simulink model "BEML_EMU"  (R2019b)
settings: configuration reference "ConfigSet_SimIntegration" (kept outside this file)
model workspace (MAT data in the model file):
  BrakesSampleTime = 0.01
  ConfigSampleTime = 0.05
  CouplingSampleTime = 0.05
  DoorsSampleTime = 0.05
  DynamicsSampleTime = 0.001
  ElectricalSampleTime = 0.05
  PRM_SimIntegration = Simulink.Parameter
  PRM_SimIntegration.Value.Dynamics.SnapToZeroVelocity = 1e-05
  PRM_SimIntegration.Value.Brakes.Equipment.AxleBrakeConfig = [1; 1; 2; 2; 0; 0]
  PRM_SimIntegration.Value.Brakes.Equipment.AxleParkBrakeConfig = [1; 2; 3; 4; 0; 0]
  PRM_SimIntegration.Value.Brakes.Equipment.NumberOfBrakeCylindersPerAxle = 2
  PRM_SimIntegration.Value.Brakes.Equipment.BrakeShoeType : enumeration (value not decoded)
  PRM_SimIntegration.Value.Brakes.BrakeCylinder.BrakeCylinderPreload = 5000
  PRM_SimIntegration.Value.Brakes.BrakeCylinder.BrakeCylinderArea = 0.024
  PRM_SimIntegration.Value.Brakes.BrakeCylinder.BrakeBeamFactor = 4.35
  PRM_SimIntegration.Value.Brakes.BrakeCylinder.BrakeEfficiency = 95
  PRM_SimIntegration.Value.Brakes.BrakeDisc.DiscBrakeRatio = 0
  PRM_SimIntegration.Value.Brakes.BrakeDisc.DiscBrakeFrictionCoef = 0
  PRM_SimIntegration.Value.Brakes.BrakeFade.BrakeTemperatures = [273; 323; 373; 423; 473; 523; 573; 623; 673; 723]
  PRM_SimIntegration.Value.Brakes.BrakeFade.BrakeEfficiencies = [1; 1; 1; 1; 1; 1; 1; 1; 1; 1]
  PRM_SimIntegration.Value.Brakes.ThermalModel.BrakeInitialTemperature = 298
  PRM_SimIntegration.Value.Brakes.ThermalModel.BrakeSpecificHeat = 500
  PRM_SimIntegration.Value.Brakes.ThermalModel.BrakeEmissivity = 0.3
  PRM_SimIntegration.Value.Brakes.ThermalModel.BrakeThermalMass = 300
  PRM_SimIntegration.Value.Brakes.ParkBrakes.ParkBrakePressures = [380000 480000]
  PRM_SimIntegration.Value.Brakes.ParkBrakes.AxleParkBrakePistonForces = [31500 0]
  PRM_SimIntegration.Value.Pneumatics.BrakeControl.LoadCompensationGains = [0.66 1]
  PRM_SimIntegration.Value.Pneumatics.BrakeControl.MaxPressure = 443000
  PRM_SimIntegration.Value.Pneumatics.MainReservoir.ResetPressure = 1000000
  PRM_SimIntegration.Value.Pneumatics.MainReservoir.MaxPressure = 1200000
  PRM_SimIntegration.Value.Pneumatics.MainReservoir.Volume = 0.2
  PRM_SimIntegration.Value.Pneumatics.MainReservoir.SwitchONPressure = 1000000
  PRM_SimIntegration.Value.Pneumatics.MainReservoir.SwitchOFFPressure = 750000
  PRM_SimIntegration.Value.Pneumatics.MainReservoir.CompressorMassFlowRate = 0.022
  PRM_SimIntegration.Value.Pneumatics.MainReservoir.BlowOffONPressure = 1050000
  PRM_SimIntegration.Value.Pneumatics.MainReservoir.BlowOffOFFPressure = 1000000
  PRM_SimIntegration.Value.Pneumatics.MainReservoirPipe.ResetPressure = 1000000
  PRM_SimIntegration.Value.Pneumatics.MainReservoirPipe.SwitchONPressure = 1000000
  PRM_SimIntegration.Value.Pneumatics.MainReservoirPipe.SwitchOFFPressure = 750000
  PRM_SimIntegration.Value.Pneumatics.Sanding.SwitchONPressure = 380000
  PRM_SimIntegration.Value.Pneumatics.Sanding.SwitchOFFPressure = 360000
  PRM_SimIntegration.Value.Pneumatics.AirSuspension.LoadCompensationMasses = [21000 33350]
  PRM_SimIntegration.Value.Pneumatics.AirSuspension.LoadCompensationPressures = [165000 440000]
  PRM_SimIntegration.Value.Pneumatics.AirSuspension.MaxPressure = 510000
  PRM_SimIntegration.Value.Pneumatics.AirSuspension.Volume = 0.07
  PRM_SimIntegration.Value.Pneumatics.AirSuspension.SwitchONPressure = 220000
  PRM_SimIntegration.Value.Pneumatics.AirSuspension.SwitchOFFPressure = 180000
  PRM_SimIntegration.Value.Pneumatics.Horn.SwitchONPressure = 140000
  PRM_SimIntegration.Value.Pneumatics.AuxiliaryReservoir.ResetPressure = 1000000
  PRM_SimIntegration.Value.Pneumatics.AuxiliaryReservoir.MaxPressure = 1000000
  PRM_SimIntegration.Value.Pneumatics.AuxiliaryReservoir.Volume = 0.025
  PRM_SimIntegration.Value.Pneumatics.AuxiliaryReservoir.SwitchONPressure = 700000
  PRM_SimIntegration.Value.Pneumatics.AuxiliaryReservoir.SwitchOFFPressure = 600000
  PRM_SimIntegration.Value.Pneumatics.AuxiliaryReservoir.CompressorMassFlowRate = 0.0014
  PRM_SimIntegration.Value.Pneumatics.AuxiliaryReservoir.BlowOffONPressure = 1020000
  PRM_SimIntegration.Value.Pneumatics.AuxiliaryReservoir.BlowOffOFFPressure = 1000000
  PRM_SimIntegration.Value.Pneumatics.Pantograph.ResetPressure = 0
  PRM_SimIntegration.Value.Pneumatics.Pantograph.MaxPressure = 1000000
  PRM_SimIntegration.Value.Pneumatics.Pantograph.Volume = 0.003
  PRM_SimIntegration.Value.Pneumatics.Pantograph.SwitchONPressure = 380000
  PRM_SimIntegration.Value.Pneumatics.Pantograph.SwitchOFFPressure = 280000
  PRM_SimIntegration.Value.Pneumatics.Pantograph.ORDSwitchONPressure = 300000
  PRM_SimIntegration.Value.Pneumatics.Pantograph.ORDSwitchOFFPressure = 240000
  PRM_SimIntegration.Value.Pneumatics.BrakeReservoir.ResetPressure = 1000000
  PRM_SimIntegration.Value.Pneumatics.BrakeReservoir.MaxPressure = 1200000
  PRM_SimIntegration.Value.Pneumatics.BrakeReservoir.Volume = 0.1
  PRM_SimIntegration.Value.Pneumatics.BrakeReservoir.SwitchONPressure = 650000
  PRM_SimIntegration.Value.Pneumatics.BrakeReservoir.SwitchOFFPressure = 550000
  PRM_SimIntegration.Value.Pneumatics.BrakeCylinder.BrakeCylindersPerBogieAxle = [2 2]
  PRM_SimIntegration.Value.Pneumatics.BrakeCylinder.ResetPressure = 0
  PRM_SimIntegration.Value.Pneumatics.BrakeCylinder.MaxPressure = 600000
  PRM_SimIntegration.Value.Pneumatics.BrakeCylinder.Volume = 0.0125
  PRM_SimIntegration.Value.Pneumatics.BrakeCylinder.SwitchONPressure = 60000
  PRM_SimIntegration.Value.Pneumatics.BrakeCylinder.SwitchOFFPressure = 30000
  PRM_SimIntegration.Value.Pneumatics.ParkBrakes.ParkBrakesPerBogieAxle = [1 1]
  PRM_SimIntegration.Value.Pneumatics.ParkBrakes.ParkBrakePressures = [300000 480000]
  PRM_SimIntegration.Value.Pneumatics.ParkBrakes.ParkBrakeForces = [31500 0]
  PRM_SimIntegration.Value.Pneumatics.ParkBrakes.SwitchONPressure = 480000
  PRM_SimIntegration.Value.Pneumatics.ParkBrakes.SwitchOFFPressure = 380000
  PRM_SimIntegration.Value.Pneumatics.VCB.ResetPressure = 0
  PRM_SimIntegration.Value.Pneumatics.VCB.MaxPressure = 1000000
  PRM_SimIntegration.Value.Pneumatics.VCB.Volume = 0.0005
  PRM_SimIntegration.Value.Pneumatics.VCB.SwitchONPressure = 435000
  PRM_SimIntegration.Value.Pneumatics.VCB.SwitchOFFPressure = 385000
  PRM_SimIntegration.Value.Traction.DesignMaxTractionTorque = 1091
  PRM_SimIntegration.Value.Traction.DesignMaxTractionPower = 210120
  PRM_SimIntegration.Value.Traction.DesignTimeToMaxTraction = 1.75
  PRM_SimIntegration.Value.Traction.DesignMaxBrakingTorque = 1570
  PRM_SimIntegration.Value.Traction.DesignMaxBrakingPower = 430000
  PRM_SimIntegration.Value.Traction.BrakeFadeRampDownSpeeds = [0.3 1]
  PRM_SimIntegration.Value.Traction.DesignGearingRatio = 6.79
  PRM_SimIntegration.Value.Traction.DesignGearingEfficiency = 0.97
  PRM_SimIntegration.Value.Traction.DesignWheelDiameter = 0.82
  PRM_SimIntegration.Value.Traction.DesignBogieMotorCount = 2
  PRM_SimIntegration.Value.Traction.AxleHasMotor = [1 1]
  PRM_SimIntegration.Value.Traction.EmergencyBrakeDeactivatesDynamicBrake = 1
  PRM_SimIntegration.Value.Traction.WheelSlipProtectionEnable = 1
  PRM_SimIntegration.Value.Traction.WheelSlideProtectionEnable = 1
  PRM_SimIntegration.Value.Traction.JerkLimit = 0.75
  PRM_SimIntegration.Value.Traction.MaxContinuousSlipBeforeTractionCutout = 10
  PRM_SimIntegration.Value.Traction.MaxContinuousSlideBeforeBrakeCutout = 10
  PRM_SimIntegration.Value.Pantograph.PantoRaiseTime = 5
  PRM_SimIntegration.Value.Pantograph.PantoLowerTime = 5
  PRM_SimIntegration.Value.Pantograph.PantoEmergencyLowerTime = 2
  PRM_SimIntegration.Value.Doors.DoorOpenTime = 2.1
  PRM_SimIntegration.Value.Doors.DoorCloseTime = 3
  PRM_SimIntegration.Value.Doors.DoorOpenAlarmTime = 5
  PRM_SimIntegration.Value.Doors.DoorCloseAlarmTime = 5
  PRM_SimIntegration.Value.Doors.DoorOpenDelay = 0.1
  PRM_SimIntegration.Value.Doors.DoorCloseDelay = 3
  PRM_SimIntegration.Value.Electrical.OverheadLineVoltage = 25000
  PRM_SimIntegration.Value.Electrical.BatteryVoltage = 110
  PRM_SimIntegration.Value.TCMS.LoadCompensationMasses = [21000 33350]
  PRM_SimIntegration.Value.TCMS.LoadCompensationPressures = [165000 440000]
  PRM_SimIntegration.Value.TCMS.TractionAccelerationTargets = [0 1.36]
  PRM_SimIntegration.Value.TCMS.BrakingDecelerationTargets = [0 1.1]
  PRM_SimIntegration.Value.TCMS.TractionBrakingDemands = [0 100]
  PRM_SimIntegration.Value.TCMS.AW3TractionAccelerationTargets = [0 1.08]
  PRM_SimIntegration.Value.TCMS.AW3BrakingDecelerationTargets = [0 0.8]
  PRM_SimIntegration.Value.Coupling.DummySignal = 0
  PRM_SimIntegration.DataType = 'Bus: BD_SimIntegration_Prm'
  PRM_SimIntegration.Dimensions = [1 1]
  PantographSampleTime = 0.05
  PneumaticsSampleTime = 0.01
  SampleTime = 0.001
  TractionSampleTime = 0.01
undefined symbols (not defined in the file): Acceleration, AngularAcceleration, AngularVelocity, BrakeFadeEnable, Brakes, BrakeShoeCoefficientCalculationMethod, BrakeShoeFrictionCoeff, BrakeTemperatureEnable, Common, DampingAdjustmentDesignMass, DavisCoeffA1, DavisCoeffA2, DavisCoeffB1, DavisCoeffB2, DavisCoefficients, DavisCoeffLeadCarC, DavisCoeffTailCarC, DiscIntNeverNeededParam, Doors, DragCalculationMethod, Dynamics, Effects, Electrical, EnableDampingAdjustmentByMass, Environment, Equipment, ExternalEffects, H, HasMotor, HasPanto, HornActivation, IsFirstVehicle, IsLastVehicle, isLeft, IsNonCab, LateralJolt, Location, LongitudinalJolt, MaxVehicles, MotionBaseSafetyCutout, OrientationDCM, P, Pantograph, Pneumatics, PneumaticsPoweredPanto, R, Traction, Transform, Tuning, UnitConfig, Velocity, VerticalJolt, VerticalJoltDown, VigilanceIntervention
libraries: simulink x35, IOStateMachinesLib x26, TestBenchLib x6, LatchesLib x3, BEML_EMU_BrakesInput_Lib x1, BEML_EMU_CBTCInterface_Lib x1, BEML_EMU_Couplers_Lib x1, BEML_EMU_DoorsInput_Lib x1, BEML_EMU_DynamicsInput_Lib x1, BEML_EMU_ElectricalInput_Lib x1, BEML_EMU_PantographInput_Lib x1, BEML_EMU_PneumaticsInput_Lib x1
(part 1 of 6)
settings Model: ParameterArgumentNames=PRM_SimIntegration  Creator=cdyer  LastModifiedBy=bnadpurohit
settings ConfigSetRef: SourceName=ConfigSet_SimIntegration  SourceLocation=Base Workspace

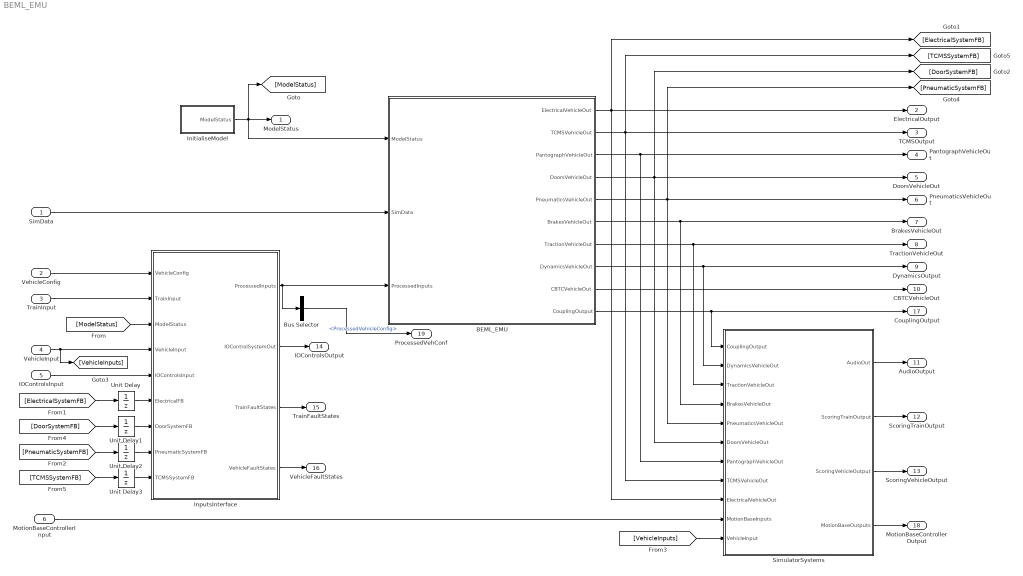
== system BEML_EMU ==
  SimData : Inport  OutDataTypeStr=Bus: BD_CommonTrain_SimulatorData  PortDimensions=1  BusOutputAsStruct=on
  VehicleConfig : Inport  Port=2  OutDataTypeStr=Bus: BD_SimIntegration_Cfg_Vehicle  PortDimensions=MaxVehicles  BusOutputAsStruct=on
  TrainInput : Inport  Port=3  OutDataTypeStr=Bus: BD_SimIntegration_In_Train  PortDimensions=1  BusOutputAsStruct=on
  VehicleInput : Inport  Port=4  OutDataTypeStr=Bus: BD_SimIntegration_In_Vehicle  PortDimensions=MaxVehicles  BusOutputAsStruct=on
  IOControlsInput : Inport  Port=5  OutDataTypeStr=Bus: BD_IOControls_In_Vehicle  PortDimensions=MaxVehicles  BusOutputAsStruct=on
  MotionBaseControllerInput : Inport  Port=6  OutDataTypeStr=Bus: BD_SimIntegration_In_Vehicle_MotionBaseController  PortDimensions=MaxVehicles  BusOutputAsStruct=on
  BEML_EMU : Subsystem
  Bus Selector : BusSelector  OutputSignals=ProcessedVehicleConfig
  InitialiseModel : Subsystem  TreatAsAtomicUnit=on  SystemSampleTime=0.5
  InputsInterface : Subsystem  TreatAsAtomicUnit=on
  SimulatorSystems : Subsystem
  Unit Delay{,1..3} (4 alike) : UnitDelay  SampleTime=-1  HasFrameUpgradeWarning=on
  ModelStatus : Outport  OutDataTypeStr=Bus: BD_CommonTrain_Out_ModelStatus  VectorParamsAs1DForOutWhenUnconnected=off  BusOutputAsStruct=on
  ElectricalOutput : Outport  Port=2  OutDataTypeStr=Bus: BD_ElectricalSystem_Out_Vehicle  VectorParamsAs1DForOutWhenUnconnected=off  BusOutputAsStruct=on
  TCMSOutput : Outport  Port=3  OutDataTypeStr=Bus: BD_TCMSSystem_Out_Vehicle  VectorParamsAs1DForOutWhenUnconnected=off  BusOutputAsStruct=on
  PantographVehicleOut : Outport  Port=4  OutDataTypeStr=Bus: BD_PantographSystem_Out_Vehicle  VectorParamsAs1DForOutWhenUnconnected=off  BusOutputAsStruct=on
  DoorsVehicleOut : Outport  Port=5  OutDataTypeStr=Bus: BD_DoorSystem_Out_Vehicle  VectorParamsAs1DForOutWhenUnconnected=off  BusOutputAsStruct=on
  PneumaticsVehicleOut : Outport  Port=6  OutDataTypeStr=Bus: BD_PneumaticsSystem_Out_Vehicle  VectorParamsAs1DForOutWhenUnconnected=off  BusOutputAsStruct=on
  BrakesVehicleOut : Outport  Port=7  OutDataTypeStr=Bus: BD_TrainBrakes_Out_Vehicle  VectorParamsAs1DForOutWhenUnconnected=off  BusOutputAsStruct=on
  TractionVehicleOut : Outport  Port=8  OutDataTypeStr=Bus: BD_TractionSystem_Out_Vehicle  VectorParamsAs1DForOutWhenUnconnected=off  BusOutputAsStruct=on
  DynamicsOutput : Outport  Port=9  OutDataTypeStr=Bus: BD_TrainDynamics_Out_Vehicle  VectorParamsAs1DForOutWhenUnconnected=off  BusOutputAsStruct=on
  CBTCVehicleOut : Outport  Port=10  OutDataTypeStr=Bus: BD_CBTC_Out_Vehicle  VectorParamsAs1DForOutWhenUnconnected=off  BusOutputAsStruct=on
  AudioOutput : Outport  Port=11  OutDataTypeStr=Bus: BD_SimIntegration_Out_Vehicle_Audio  VectorParamsAs1DForOutWhenUnconnected=off  BusOutputAsStruct=on
  "ScoringTrainOutput " : Outport  Port=12  OutDataTypeStr=Bus: BD_SimIntegration_Out_Train_Scoring  VectorParamsAs1DForOutWhenUnconnected=off  BusOutputAsStruct=on
  ScoringVehicleOutput : Outport  Port=13  OutDataTypeStr=Bus: BD_SimIntegration_Out_Vehicle_Scoring  VectorParamsAs1DForOutWhenUnconnected=off  BusOutputAsStruct=on
  IOControlsOutput : Outport  Port=14  OutDataTypeStr=Bus: BD_IOControls_Out_Vehicle  VectorParamsAs1DForOutWhenUnconnected=off  BusOutputAsStruct=on
  TrainFaultStates : Outport  Port=15  OutDataTypeStr=Bus: BD_SimIntegration_Faults_Train  VectorParamsAs1DForOutWhenUnconnected=off  LockScale=on  BusOutputAsStruct=on
  VehicleFaultStates : Outport  Port=16  OutDataTypeStr=Bus: BD_SimIntegration_Faults_Vehicle  VectorParamsAs1DForOutWhenUnconnected=off  BusOutputAsStruct=on
  CouplingOutput : Outport  Port=17  OutDataTypeStr=Bus: BD_CouplingSystem_Out_Vehicle  VectorParamsAs1DForOutWhenUnconnected=off  BusOutputAsStruct=on
  MotionBaseControllerOutput : Outport  Port=18  OutDataTypeStr=Bus: BD_SimIntegration_Out_Vehicle_MotionBaseController  VectorParamsAs1DForOutWhenUnconnected=off  BusOutputAsStruct=on
  ProcessedVehConf : Outport  Port=19  OutDataTypeStr=Bus: BD_SimIntegration_Cfg_Vehicle  VectorParamsAs1DForOutWhenUnconnected=off  BusOutputAsStruct=on
  wires:
  VehicleConfig/1 -> InputsInterface/1(VehicleConfig)
  TrainInput/1 -> InputsInterface/2(TrainInput)
  VehicleInput/1 -> [VehicleInputs], InputsInterface/4(VehicleInput)
  IOControlsInput/1 -> InputsInterface/5(IOControlsInput)
  InputsInterface/4(VehicleFaultStates) -> VehicleFaultStates/1
  InputsInterface/3(TrainFaultStates) -> TrainFaultStates/1
  InputsInterface/2(IOControlSystemOut) -> IOControlsOutput/1
  SimData/1 -> BEML_EMU/2(SimData)
  BEML_EMU/8(DynamicsVehicleOut) -> DynamicsOutput/1, SimulatorSystems/2(DynamicsVehicleOut)
  InitialiseModel/1(ModelStatus) -> [ModelStatus], BEML_EMU/1(ModelStatus), ModelStatus/1
  SimulatorSystems/1(AudioOut) -> AudioOutput/1
  SimulatorSystems/2(ScoringTrainOutput) -> "ScoringTrainOutput "/1
  SimulatorSystems/3(ScoringVehicleOutput) -> ScoringVehicleOutput/1
  InputsInterface/1(ProcessedInputs) -> Bus Selector/1, BEML_EMU/3(ProcessedInputs)
  BEML_EMU/5(PneumaticsVehicleOut) -> PneumaticsVehicleOut/1, [PneumaticSystemFB], SimulatorSystems/5(PneumaticsVehicleOut)
  BEML_EMU/3(PantographVehicleOut) -> PantographVehicleOut/1, SimulatorSystems/7(PantographVehicleOut)
  BEML_EMU/7(TractionVehicleOut) -> TractionVehicleOut/1, SimulatorSystems/3(TractionVehicleOut)
  BEML_EMU/6(BrakesVehicleOut) -> BrakesVehicleOut/1, SimulatorSystems/4(BrakesVehicleOut)
  BEML_EMU/4(DoorsVehicleOut) -> DoorsVehicleOut/1, [DoorSystemFB], SimulatorSystems/6(DoorsVehicleOut)
  BEML_EMU/2(TCMSVehicleOut) -> TCMSOutput/1, [TCMSSystemFB], SimulatorSystems/8(TCMSVehicleOut)
  BEML_EMU/1(ElectricalVehicleOut) -> ElectricalOutput/1, [ElectricalSystemFB], SimulatorSystems/9(ElectricalVehicleOut)
  BEML_EMU/9(CBTCVehicleOut) -> CBTCVehicleOut/1
  [ModelStatus] -> InputsInterface/3(ModelStatus)
  BEML_EMU/10(CouplingOutput) -> CouplingOutput/1, SimulatorSystems/1(CouplingOutput)
  SimulatorSystems/4(MotionBaseOutputs) -> MotionBaseControllerOutput/1
  MotionBaseControllerInput/1 -> SimulatorSystems/10(MotionBaseInputs)
  [ElectricalSystemFB] -> Unit Delay/1
  Unit Delay/1 -> InputsInterface/6(ElectricalFB)
  [VehicleInputs] -> SimulatorSystems/11(VehicleInput)
  [DoorSystemFB] -> Unit Delay1/1
  Unit Delay1/1 -> InputsInterface/7(DoorSystemFB)
  Bus Selector/1 -> ProcessedVehConf/1  "<ProcessedVehicleConfig>"
  [PneumaticSystemFB] -> Unit Delay2/1
  Unit Delay2/1 -> InputsInterface/8(PneumaticSystemFB)
  Unit Delay3/1 -> InputsInterface/9(TCMSSystemFB)
  [TCMSSystemFB] -> Unit Delay3/1

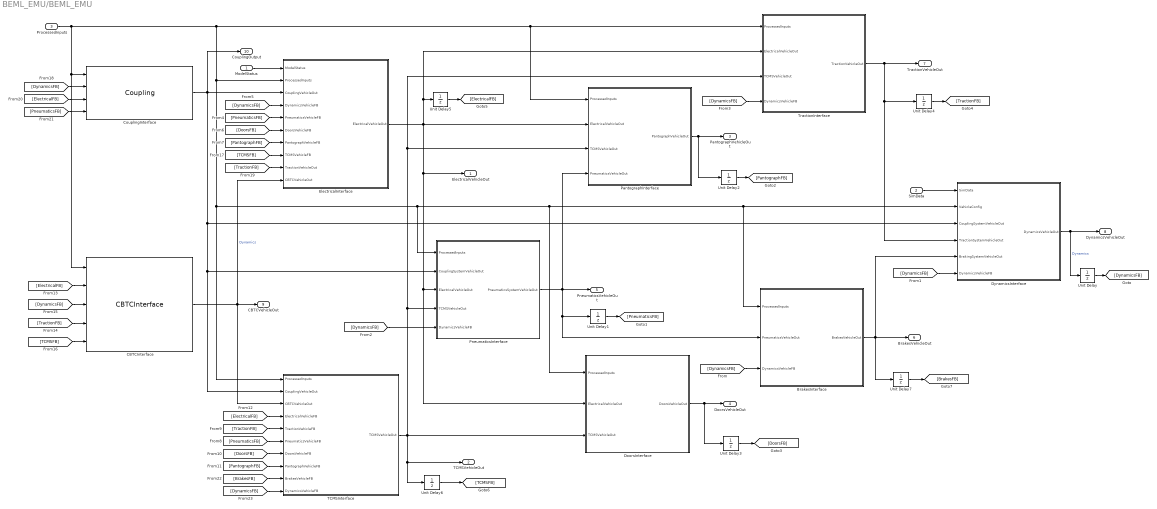
== system BEML_EMU/BEML_EMU ==
  ModelStatus : Inport
  SimData : Inport  Port=2
  ProcessedInputs : Inport  Port=3
  BrakesInterface : Subsystem  SystemSampleTime=0.001
      mask Display: disp("Brakes");
  CBTCInterface : BEML_EMU_CBTCInterface_Lib/CBTCInterface  SystemSampleTime=0.001  Latency=0  AutoFrameSizeCalculation=off
      mask Display:
      | % This is a new mask on top of the base mask.
      | % Use "View base mask" link below to see the base mask.
      | disp("CBTC");
  CouplingInterface : BEML_EMU_Couplers_Lib/Coupling  SystemSampleTime=CouplingSampleTime  Latency=0  AutoFrameSizeCalculation=off
      mask Display:
      | % This is a new mask on top of the base mask.
      | % Use "View base mask" link below to see the base mask.
      | disp("Coupling");
  DoorsInterface : Subsystem  SystemSampleTime=0.001
      mask Display: disp("Doors");
  DynamicsInterface : Subsystem  SystemSampleTime=0.001
      mask Display: disp("Dynamics");
  ElectricalInterface : Subsystem  SystemSampleTime=0.001
      mask Display: disp("Electrical");
  PantographInterface : Subsystem  SystemSampleTime=0.001
      mask Display: disp("Pantograph");
  PneumaticsInterface : Subsystem  SystemSampleTime=0.001
      mask Display: disp("Pneumatics");
  TCMSInterface : Subsystem  SystemSampleTime=0.001
      mask Display: disp("TCMS");
  TractionInterface : Subsystem  SystemSampleTime=0.001
      mask Display: disp("Traction");
  Unit Delay{,1..7} (8 alike) : UnitDelay  SampleTime=-1  HasFrameUpgradeWarning=on
  ElectricalVehicleOut : Outport  VectorParamsAs1DForOutWhenUnconnected=off
  TCMSVehicleOut : Outport  Port=2  VectorParamsAs1DForOutWhenUnconnected=off
  PantographVehicleOut : Outport  Port=3  VectorParamsAs1DForOutWhenUnconnected=off
  DoorsVehicleOut : Outport  Port=4  VectorParamsAs1DForOutWhenUnconnected=off
  PneumaticsVehicleOut : Outport  Port=5  VectorParamsAs1DForOutWhenUnconnected=off
  BrakesVehicleOut : Outport  Port=6  VectorParamsAs1DForOutWhenUnconnected=off
  TractionVehicleOut : Outport  Port=7  VectorParamsAs1DForOutWhenUnconnected=off
  DynamicsVehicleOut : Outport  Port=8  VectorParamsAs1DForOutWhenUnconnected=off
  CBTCVehicleOut : Outport  Port=9  VectorParamsAs1DForOutWhenUnconnected=off
  CouplingOutput : Outport  Port=10  VectorParamsAs1DForOutWhenUnconnected=off
  wires:
  SimData/1 -> DynamicsInterface/1(SimData)
  DynamicsInterface/1(DynamicsVehicleOut) -> DynamicsVehicleOut/1, Unit Delay/1  "Dynamics"
  Unit Delay/1 -> [DynamicsFB]
  [DynamicsFB] -> BrakesInterface/3(DynamicsVehicleFB)
  [DynamicsFB] -> DynamicsInterface/6(DynamicsVehicleFB)
  PneumaticsInterface/1(PneumaticsSystemVehicleOut) -> PantographInterface/4(PneumaticsVehicleOut), PneumaticsVehicleOut/1, Unit Delay1/1, BrakesInterface/2(PneumaticsVehicleOut)
  ProcessedInputs/1 -> CBTCInterface/1, CouplingInterface/1, PantographInterface/1(ProcessedInputs), TractionInterface/1(ProcessedInputs), DoorsInterface/1(ProcessedInputs), DynamicsInterface/2(VehicleConfig), BrakesInterface/1(ProcessedInputs), PneumaticsInterface/1(ProcessedInputs), TCMSInterface/1(ProcessedInputs), ElectricalInterface/2(ProcessedInputs)
  CouplingInterface/1 -> DynamicsInterface/3(CouplingSystemVehicleOut), PneumaticsInterface/2(CouplingSystemVehicleOut), TCMSInterface/2(CouplingVehicleOut), CouplingOutput/1, ElectricalInterface/3(CouplingVehicleOut)
  [DynamicsFB] -> PneumaticsInterface/5(DynamicsVehicleFB)
  ElectricalInterface/1(ElectricalVehicleOut) -> ElectricalVehicleOut/1, PneumaticsInterface/3(ElectricalVehicleOut), DoorsInterface/2(ElectricalVehicleOut), PantographInterface/2(ElectricalVehicleOut), Unit Delay5/1, TractionInterface/2(ElectricalVehicleOut)
  [DynamicsFB] -> TractionInterface/4(DynamicsVehicleFB)
  TCMSInterface/1(TCMSVehicleOut) -> Unit Delay6/1, TCMSVehicleOut/1, TractionInterface/3(TCMSVehicleOut), PantographInterface/3(TCMSVehicleOut), PneumaticsInterface/4(TCMSVehicleOut), DoorsInterface/3(TCMSVehicleOut)
  PantographInterface/1(PantographVehicleOut) -> Unit Delay2/1, PantographVehicleOut/1
  DoorsInterface/1(DoorsVehicleOut) -> Unit Delay3/1, DoorsVehicleOut/1
  TractionInterface/1(TractionVehicleOut) -> TractionVehicleOut/1, Unit Delay4/1, DynamicsInterface/4(TractionSystemVehicleOut)
  Unit Delay1/1 -> [PneumaticsFB]
  [PneumaticsFB] -> ElectricalInterface/5(PneumaticsVehicleFB)
  [DynamicsFB] -> ElectricalInterface/4(DynamicsVehicleFB)
  Unit Delay2/1 -> [PantographFB]
  Unit Delay3/1 -> [DoorsFB]
  [DoorsFB] -> ElectricalInterface/6(DoorsVehicleFB)
  [PantographFB] -> ElectricalInterface/7(PantographVehicleFB)
  ModelStatus/1 -> ElectricalInterface/1(ModelStatus)
  [PantographFB] -> TCMSInterface/8(PantographVehicleFB)
  [DoorsFB] -> TCMSInterface/7(DoorsVehicleFB)
  [TractionFB] -> TCMSInterface/5(TractionVehicleFB)
  [PneumaticsFB] -> TCMSInterface/6(PneumaticsVehicleFB)
  Unit Delay4/1 -> [TractionFB]
  Unit Delay5/1 -> [ElectricalFB]
  [ElectricalFB] -> TCMSInterface/4(ElectricalVehicleFB)
  [ElectricalFB] -> CBTCInterface/2
  [TractionFB] -> CBTCInterface/4
  [DynamicsFB] -> CBTCInterface/3
  [TCMSFB] -> CBTCInterface/5
  CBTCInterface/1 -> ElectricalInterface/10(CBTCVehicleOut), TCMSInterface/3(CBTCVehicleOut), CBTCVehicleOut/1  "Dynamics"
  Unit Delay6/1 -> [TCMSFB]
  [TCMSFB] -> ElectricalInterface/8(TCMSVehicleFB)
  [DynamicsFB] -> CouplingInterface/2
  [ElectricalFB] -> CouplingInterface/3
  [PneumaticsFB] -> CouplingInterface/4
  Unit Delay7/1 -> [BrakesFB]
  BrakesInterface/1(BrakesVehicleOut) -> Unit Delay7/1, DynamicsInterface/5(BrakingSystemVehicleOut), BrakesVehicleOut/1
  [BrakesFB] -> TCMSInterface/9(BrakesVehicleFB)
  [TractionFB] -> ElectricalInterface/9(TractionVehicleOut)
  [DynamicsFB] -> TCMSInterface/10(DynamicsVehicleFB)

== system BEML_EMU/InitialiseModel ==
  Bus Creator : BusCreator  Inputs=1  OutDataTypeStr=Bus: BD_CommonTrain_Out_ModelStatus  NonVirtualBus=on
      settings: InheritFromInputs=off
  Step : Step  Time=2
  double to boolean : DataTypeConversion
  ModelStatus : Outport  VectorParamsAs1DForOutWhenUnconnected=off
  wires:
  Bus Creator/1 -> ModelStatus/1
  Step/1 -> double to boolean/1
  double to boolean/1 -> Bus Creator/1  "IsInitialized"

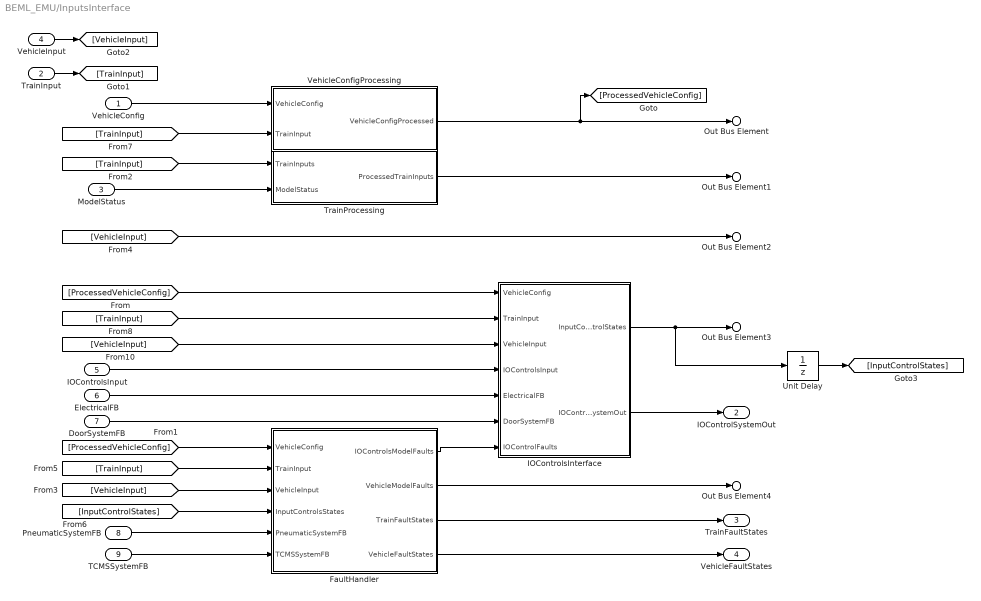
== system BEML_EMU/InputsInterface ==
  VehicleConfig : Inport
  TrainInput : Inport  Port=2
  ModelStatus : Inport  Port=3
  VehicleInput : Inport  Port=4
  IOControlsInput : Inport  Port=5
  ElectricalFB : Inport  Port=6
  DoorSystemFB : Inport  Port=7
  PneumaticSystemFB : Inport  Port=8
  TCMSSystemFB : Inport  Port=9
  FaultHandler : Subsystem
  IOControlsInterface : Subsystem
  TrainProcessing : Subsystem
  Unit Delay : UnitDelay  SampleTime=-1  HasFrameUpgradeWarning=on
  VehicleConfigProcessing : Subsystem  TreatAsAtomicUnit=on  SystemSampleTime=ConfigSampleTime
  Out Bus Element : Outport  PortName=ProcessedInputs  Element=ProcessedVehicleConfig
  Out Bus Element1 : Outport  PortName=ProcessedInputs  Element=ProcessedTrainInput
  Out Bus Element2 : Outport  PortName=ProcessedInputs  Element=ProcessedVehicleInput
  Out Bus Element3 : Outport  PortName=ProcessedInputs  Element=InputControlStates
  Out Bus Element4 : Outport  PortName=ProcessedInputs  Element=VehicleModelFaults
  IOControlSystemOut : Outport  Port=2  VectorParamsAs1DForOutWhenUnconnected=off
  TrainFaultStates : Outport  Port=3  VectorParamsAs1DForOutWhenUnconnected=off
  VehicleFaultStates : Outport  Port=4  VectorParamsAs1DForOutWhenUnconnected=off
  wires:
  VehicleInput/1 -> [VehicleInput]
  TrainInput/1 -> [TrainInput]
  [ProcessedVehicleConfig] -> IOControlsInterface/1(VehicleConfig)
  IOControlsInput/1 -> IOControlsInterface/4(IOControlsInput)
  IOControlsInterface/1(InputControlStates) -> Out Bus Element3/1, Unit Delay/1
  IOControlsInterface/2(IOControlSystemOut) -> IOControlSystemOut/1
  VehicleConfig/1 -> VehicleConfigProcessing/1(VehicleConfig)
  [TrainInput] -> IOControlsInterface/2(TrainInput)
  [VehicleInput] -> IOControlsInterface/3(VehicleInput)
  [VehicleInput] -> Out Bus Element2/1
  [ProcessedVehicleConfig] -> FaultHandler/1(VehicleConfig)
  [TrainInput] -> FaultHandler/2(TrainInput)
  [VehicleInput] -> FaultHandler/3(VehicleInput)
  FaultHandler/3(TrainFaultStates) -> TrainFaultStates/1
  FaultHandler/4(VehicleFaultStates) -> VehicleFaultStates/1
  FaultHandler/2(VehicleModelFaults) -> Out Bus Element4/1
  [InputControlStates] -> FaultHandler/4(InputControlsStates)
  Unit Delay/1 -> [InputControlStates]
  FaultHandler/1(IOControlsModelFaults) -> IOControlsInterface/7(IOControlFaults)
  VehicleConfigProcessing/1(VehicleConfigProcessed) -> [ProcessedVehicleConfig], Out Bus Element/1
  [TrainInput] -> VehicleConfigProcessing/2(TrainInput)
  [TrainInput] -> TrainProcessing/1(TrainInputs)
  TrainProcessing/1(ProcessedTrainInputs) -> Out Bus Element1/1
  ModelStatus/1 -> TrainProcessing/2(ModelStatus)
  ElectricalFB/1 -> IOControlsInterface/5(ElectricalFB)
  DoorSystemFB/1 -> IOControlsInterface/6(DoorSystemFB)
  PneumaticSystemFB/1 -> FaultHandler/5(PneumaticSystemFB)
  TCMSSystemFB/1 -> FaultHandler/6(TCMSSystemFB)

== system BEML_EMU/SimulatorSystems ==
  note: Things like
      | Audio logic
      | Motion Base Adapter
      | Vision output logic
      | Scripting Triggers
      | Reporting Values
      | Special Display Application Values
  CouplingOutput : Inport
  DynamicsVehicleOut : Inport  Port=2
  TractionVehicleOut : Inport  Port=3
  BrakesVehicleOut : Inport  Port=4
  PneumaticsVehicleOut : Inport  Port=5
  DoorsVehicleOut : Inport  Port=6
  PantographVehicleOut : Inport  Port=7
  TCMSVehicleOut : Inport  Port=8
  ElectricalVehicleOut : Inport  Port=9
  MotionBaseInputs : Inport  Port=10
  VehicleInput : Inport  Port=11
  AudioSystemInterface : Subsystem  TreatAsAtomicUnit=on  SystemSampleTime=ConfigSampleTime
  Dynamics : Subsystem
  ScoringSystemInterface : Subsystem  TreatAsAtomicUnit=on  SystemSampleTime=ConfigSampleTime
  Subsystem : Subsystem
  AudioOut : Outport  VectorParamsAs1DForOutWhenUnconnected=off
  ScoringTrainOutput : Outport  Port=2  VectorParamsAs1DForOutWhenUnconnected=off
  ScoringVehicleOutput : Outport  Port=3  VectorParamsAs1DForOutWhenUnconnected=off  BusOutputAsStruct=on
  MotionBaseOutputs : Outport  Port=4
  wires:
  DynamicsVehicleOut/1 -> Subsystem/3(DynamicsVehicleOut), ScoringSystemInterface/1(DynamicsVehicleOut), AudioSystemInterface/1(DynamicsVehicleOut1)
  AudioSystemInterface/1(AudioOut) -> AudioOut/1
  ScoringSystemInterface/1(ScoringTrainOutput) -> ScoringTrainOutput/1
  ScoringSystemInterface/2(ScoringVehicleOutputs) -> ScoringVehicleOutput/1
  TractionVehicleOut/1 -> ScoringSystemInterface/2(TractionVehicleOut), AudioSystemInterface/2(TractionVehicleOut1)
  BrakesVehicleOut/1 -> ScoringSystemInterface/3(BrakesVehicleOut), AudioSystemInterface/3(BrakesVehicleOut1)
  PneumaticsVehicleOut/1 -> ScoringSystemInterface/4(PneumaticsVehicleOut), AudioSystemInterface/4(PneumaticsVehicleOut1)
  DoorsVehicleOut/1 -> ScoringSystemInterface/5(DoorsVehicleOut), AudioSystemInterface/5(DoorsVehicleOut1)
  PantographVehicleOut/1 -> ScoringSystemInterface/6(PantographVehicleOut), AudioSystemInterface/6(PantographVehicleOut1)
  TCMSVehicleOut/1 -> ScoringSystemInterface/7(TCMSVehicleOut), AudioSystemInterface/7(TCMSVehicleOut1)
  ElectricalVehicleOut/1 -> ScoringSystemInterface/8(ElectricalVehicleOut), AudioSystemInterface/8(ElectricalVehicleOut1)
  CouplingOutput/1 -> AudioSystemInterface/9(CouplingOutput)
  MotionBaseInputs/1 -> Subsystem/4(MotionBase Inputs)
  VehicleInput/1 -> Dynamics/1(VehicleIn), Subsystem/1(Vehicle Input)
  Subsystem/1(MotionBaseOutputs) -> MotionBaseOutputs/1
  Dynamics/1(<Dynamics>) -> Subsystem/2(Dynamics Input)

== system BEML_EMU/BEML_EMU/BrakesInterface ==
  In Bus Element : Inport  PortName=ProcessedInputs  Element=ProcessedVehicleConfig
  In Bus Element1 : Inport  PortName=ProcessedInputs  Element=ProcessedTrainInput
  In Bus Element2 : Inport  PortName=ProcessedInputs  Element=ProcessedVehicleInput
  In Bus Element4 : Inport  PortName=ProcessedInputs  Element=VehicleModelFaults
  PneumaticsVehicleOut : Inport  Port=2
  DynamicsVehicleFB : Inport  Port=3
  BrakesInputAdapter : BEML_EMU_BrakesInput_Lib/BrakesInputAdapter  SystemSampleTime=BrakesSampleTime  Latency=0  AutoFrameSizeCalculation=off
  TrainBrakes : ModelReference  ModelNameDialog=TrainBrakes  ParameterArgumentNames=PRM_TrainBrakes_Vehicles  ParameterArgumentValues=PRM_SimIntegration.Brakes  UsingDefaultArgumentValue=0  SimulationMode=Normal  ModelReferenceVersion=1.18
  BrakesVehicleOut : Outport  VectorParamsAs1DForOutWhenUnconnected=off
  wires:
  In Bus Element1/1 -> BrakesInputAdapter/2
  In Bus Element2/1 -> BrakesInputAdapter/3
  In Bus Element4/1 -> BrakesInputAdapter/4
  BrakesInputAdapter/3 -> TrainBrakes/3
  In Bus Element/1 -> BrakesInputAdapter/1
  BrakesInputAdapter/1 -> TrainBrakes/1
  BrakesInputAdapter/5 -> TrainBrakes/5
  BrakesInputAdapter/4 -> TrainBrakes/4
  BrakesInputAdapter/2 -> TrainBrakes/2
  DynamicsVehicleFB/1 -> BrakesInputAdapter/6
  PneumaticsVehicleOut/1 -> BrakesInputAdapter/5
  TrainBrakes/1 -> BrakesVehicleOut/1

== system BEML_EMU/BEML_EMU/DoorsInterface ==
  In Bus Element : Inport  PortName=ProcessedInputs  Element=ProcessedVehicleConfig
  In Bus Element1 : Inport  PortName=ProcessedInputs  Element=ProcessedTrainInput
  In Bus Element2 : Inport  PortName=ProcessedInputs  Element=ProcessedVehicleInput
  In Bus Element4 : Inport  PortName=ProcessedInputs  Element=VehicleModelFaults
  In Bus Element3 : Inport  PortName=ProcessedInputs  Element=InputControlStates
  ElectricalVehicleOut : Inport  Port=2
  TCMSVehicleOut : Inport  Port=3
  DoorsInputAdapter : BEML_EMU_DoorsInput_Lib/DoorsInterface/DoorsInputAdapter  SystemSampleTime=DoorsSampleTime  Latency=0  AutoFrameSizeCalculation=off
  DoorsSystem : ModelReference  ModelNameDialog=DoorSystem  ParameterArgumentNames=PRM_DoorSystem  ParameterArgumentValues=PRM_SimIntegration.Doors  UsingDefaultArgumentValue=0  SimulationMode=Normal  ModelReferenceVersion=1.2208
  DoorsVehicleOut : Outport  VectorParamsAs1DForOutWhenUnconnected=off
  wires:
  DoorsSystem/1 -> DoorsVehicleOut/1
  ElectricalVehicleOut/1 -> DoorsInputAdapter/6
  DoorsInputAdapter/1 -> DoorsSystem/1
  In Bus Element/1 -> DoorsInputAdapter/1
  In Bus Element4/1 -> DoorsInputAdapter/5
  In Bus Element2/1 -> DoorsInputAdapter/3
  In Bus Element1/1 -> DoorsInputAdapter/2
  TCMSVehicleOut/1 -> DoorsInputAdapter/7
  In Bus Element3/1 -> DoorsInputAdapter/4
  DoorsInputAdapter/2 -> DoorsSystem/2
  DoorsInputAdapter/3 -> DoorsSystem/3
  DoorsInputAdapter/4 -> DoorsSystem/4

== system BEML_EMU/BEML_EMU/DynamicsInterface ==
  SimData : Inport
  In Bus Element : Inport  Port=2  PortName=VehicleConfig  Element=ProcessedVehicleConfig
  In Bus Element1 : Inport  Port=2  PortName=VehicleConfig  Element=ProcessedTrainInput
  In Bus Element2 : Inport  Port=2  PortName=VehicleConfig  Element=ProcessedVehicleInput
  In Bus Element4 : Inport  Port=2  PortName=VehicleConfig  Element=VehicleModelFaults
  CouplingSystemVehicleOut : Inport  Port=3
  TractionSystemVehicleOut : Inport  Port=4
  BrakingSystemVehicleOut : Inport  Port=5
  DynamicsVehicleFB : Inport  Port=6
  DynamicsInputAdapter : BEML_EMU_DynamicsInput_Lib/DynamicsInputAdapter  SystemSampleTime=DynamicsSampleTime  Latency=0  AutoFrameSizeCalculation=off
  TrainDynamics : ModelReference  ModelNameDialog=TrainDynamics  ParameterArgumentNames=Prm_TrainDynamics  ParameterArgumentValues=PRM_SimIntegration.Dynamics  UsingDefaultArgumentValue=0  SimulationMode=Normal  ModelReferenceVersion=1.791
  DynamicsVehicleOut : Outport  VectorParamsAs1DForOutWhenUnconnected=off
  wires:
  TrainDynamics/1 -> DynamicsVehicleOut/1
  TractionSystemVehicleOut/1 -> DynamicsInputAdapter/5
  BrakingSystemVehicleOut/1 -> DynamicsInputAdapter/6
  DynamicsInputAdapter/2 -> TrainDynamics/3
  DynamicsInputAdapter/4 -> TrainDynamics/5
  DynamicsInputAdapter/5 -> TrainDynamics/6
  DynamicsInputAdapter/1 -> TrainDynamics/2
  In Bus Element/1 -> DynamicsInputAdapter/1
  DynamicsInputAdapter/3 -> TrainDynamics/4
  In Bus Element4/1 -> DynamicsInputAdapter/4
  In Bus Element2/1 -> DynamicsInputAdapter/3
  In Bus Element1/1 -> DynamicsInputAdapter/2
  SimData/1 -> TrainDynamics/1
  DynamicsVehicleFB/1 -> DynamicsInputAdapter/8
  CouplingSystemVehicleOut/1 -> DynamicsInputAdapter/7

== system BEML_EMU/BEML_EMU/ElectricalInterface ==
  ModelStatus : Inport
  In Bus Element : Inport  Port=2  PortName=ProcessedInputs  Element=ProcessedVehicleConfig
  In Bus Element1 : Inport  Port=2  PortName=ProcessedInputs  Element=ProcessedTrainInput
  In Bus Element2 : Inport  Port=2  PortName=ProcessedInputs  Element=ProcessedVehicleInput
  In Bus Element4 : Inport  Port=2  PortName=ProcessedInputs  Element=VehicleModelFaults
  In Bus Element3 : Inport  Port=2  PortName=ProcessedInputs  Element=InputControlStates
  CouplingVehicleOut : Inport  Port=3
  DynamicsVehicleFB : Inport  Port=4
  PneumaticsVehicleFB : Inport  Port=5
  DoorsVehicleFB : Inport  Port=6
  PantographVehicleFB : Inport  Port=7
  TCMSVehicleFB : Inport  Port=8
  TractionVehicleOut : Inport  Port=9
  CBTCVehicleOut : Inport  Port=10
  ElectricalInputAdapter : BEML_EMU_ElectricalInput_Lib/ElectricalInputAdapter  SystemSampleTime=ElectricalSampleTime  Latency=0  AutoFrameSizeCalculation=off
  ElectricalSystem : ModelReference  ModelNameDialog=ElectricalSystem  ParameterArgumentNames=Prm_ElectricalSystem  ParameterArgumentValues=PRM_SimIntegration.Electrical  UsingDefaultArgumentValue=0  SimulationMode=Normal  ModelReferenceVersion=1.2061
  Terminator : Terminator
  ElectricalVehicleOut : Outport  VectorParamsAs1DForOutWhenUnconnected=off
  wires:
  ElectricalSystem/1 -> ElectricalVehicleOut/1
  CouplingVehicleOut/1 -> ElectricalInputAdapter/7
  PneumaticsVehicleFB/1 -> ElectricalInputAdapter/9
  ElectricalInputAdapter/2 -> ElectricalSystem/2
  ElectricalInputAdapter/4 -> ElectricalSystem/4
  ElectricalInputAdapter/5 -> ElectricalSystem/5
  ElectricalInputAdapter/1 -> ElectricalSystem/1
  In Bus Element/1 -> ElectricalInputAdapter/2
  ElectricalInputAdapter/3 -> ElectricalSystem/3
  In Bus Element4/1 -> ElectricalInputAdapter/6
  In Bus Element2/1 -> ElectricalInputAdapter/4
  In Bus Element1/1 -> ElectricalInputAdapter/3
  DynamicsVehicleFB/1 -> ElectricalInputAdapter/8
  In Bus Element3/1 -> ElectricalInputAdapter/5
  DoorsVehicleFB/1 -> ElectricalInputAdapter/10
  PantographVehicleFB/1 -> ElectricalInputAdapter/11
  ElectricalSystem/2 -> Terminator/1
  ModelStatus/1 -> ElectricalInputAdapter/1
  TCMSVehicleFB/1 -> ElectricalInputAdapter/12
  CBTCVehicleOut/1 -> ElectricalInputAdapter/14
  TractionVehicleOut/1 -> ElectricalInputAdapter/13

== system BEML_EMU/BEML_EMU/PantographInterface ==
  In Bus Element : Inport  PortName=ProcessedInputs  Element=ProcessedVehicleConfig
  In Bus Element1 : Inport  PortName=ProcessedInputs  Element=ProcessedTrainInput
  In Bus Element2 : Inport  PortName=ProcessedInputs  Element=ProcessedVehicleInput
  In Bus Element4 : Inport  PortName=ProcessedInputs  Element=VehicleModelFaults
  ElectricalVehicleOut : Inport  Port=2
  TCMSVehicleOut : Inport  Port=3
  PneumaticsVehicleOut : Inport  Port=4
  PantographInputAdapter : BEML_EMU_PantographInput_Lib/PantographInputAdapter  SystemSampleTime=PantographSampleTime  Latency=0  AutoFrameSizeCalculation=off
  PantographSystem : ModelReference  ModelNameDialog=PantographSystem  ParameterArgumentNames=Prm_PantographSystem  ParameterArgumentValues=PRM_SimIntegration.Pantograph  UsingDefaultArgumentValue=0  SimulationMode=Normal  ModelReferenceVersion=1.936
  PantographVehicleOut : Outport  VectorParamsAs1DForOutWhenUnconnected=off
  wires:
  TCMSVehicleOut/1 -> PantographInputAdapter/6
  In Bus Element1/1 -> PantographInputAdapter/2
  In Bus Element2/1 -> PantographInputAdapter/3
  In Bus Element4/1 -> PantographInputAdapter/4
  PantographInputAdapter/3 -> PantographSystem/3
  In Bus Element/1 -> PantographInputAdapter/1
  PantographInputAdapter/1 -> PantographSystem/1
  PantographInputAdapter/5 -> PantographSystem/5
  PantographInputAdapter/4 -> PantographSystem/4
  PantographInputAdapter/2 -> PantographSystem/2
  PneumaticsVehicleOut/1 -> PantographInputAdapter/7
  ElectricalVehicleOut/1 -> PantographInputAdapter/5
  PantographSystem/1 -> PantographVehicleOut/1

== system BEML_EMU/BEML_EMU/PneumaticsInterface ==
  In Bus Element : Inport  PortName=ProcessedInputs  Element=ProcessedVehicleConfig
  In Bus Element1 : Inport  PortName=ProcessedInputs  Element=ProcessedTrainInput
  In Bus Element2 : Inport  PortName=ProcessedInputs  Element=ProcessedVehicleInput
  In Bus Element4 : Inport  PortName=ProcessedInputs  Element=VehicleModelFaults
  In Bus Element3 : Inport  PortName=ProcessedInputs  Element=InputControlStates
  CouplingSystemVehicleOut : Inport  Port=2
  ElectricalVehicleOut : Inport  Port=3
  TCMSVehicleOut : Inport  Port=4
  DynamicsVehicleFB : Inport  Port=5
  PneumaticsInputAdapter : BEML_EMU_PneumaticsInput_Lib/PneumaticsInputAdapter  SystemSampleTime=PneumaticsSampleTime  Latency=0  AutoFrameSizeCalculation=off
  PneumaticsSystem : ModelReference  ModelNameDialog=PneumaticsSystem  ParameterArgumentNames=Prm_PneumaticsSystem  ParameterArgumentValues=PRM_SimIntegration.Pneumatics  UsingDefaultArgumentValue=0  SimulationMode=Normal  ModelReferenceVersion=1.664
  PneumaticsSystemVehicleOut : Outport  VectorParamsAs1DForOutWhenUnconnected=off
  wires:
  PneumaticsSystem/1 -> PneumaticsSystemVehicleOut/1
  ElectricalVehicleOut/1 -> PneumaticsInputAdapter/6
  DynamicsVehicleFB/1 -> PneumaticsInputAdapter/9
  PneumaticsInputAdapter/2 -> PneumaticsSystem/2
  PneumaticsInputAdapter/4 -> PneumaticsSystem/4
  PneumaticsInputAdapter/5 -> PneumaticsSystem/5
  PneumaticsInputAdapter/1 -> PneumaticsSystem/1
  In Bus Element/1 -> PneumaticsInputAdapter/1
  PneumaticsInputAdapter/3 -> PneumaticsSystem/3
  In Bus Element4/1 -> PneumaticsInputAdapter/5
  In Bus Element2/1 -> PneumaticsInputAdapter/3
  In Bus Element1/1 -> PneumaticsInputAdapter/2
  CouplingSystemVehicleOut/1 -> PneumaticsInputAdapter/8
  In Bus Element3/1 -> PneumaticsInputAdapter/4
  TCMSVehicleOut/1 -> PneumaticsInputAdapter/7

== system BEML_EMU/BEML_EMU/TCMSInterface ==
  In Bus Element : Inport  PortName=ProcessedInputs  Element=ProcessedVehicleConfig
  In Bus Element1 : Inport  PortName=ProcessedInputs  Element=ProcessedTrainInput
  In Bus Element2 : Inport  PortName=ProcessedInputs  Element=ProcessedVehicleInput
  In Bus Element4 : Inport  PortName=ProcessedInputs  Element=VehicleModelFaults
  In Bus Element3 : Inport  PortName=ProcessedInputs  Element=InputControlStates
  CouplingVehicleOut : Inport  Port=2
  CBTCVehicleOut : Inport  Port=3
  ElectricalVehicleFB : Inport  Port=4
  TractionVehicleFB : Inport  Port=5
  PneumaticsVehicleFB : Inport  Port=6
  DoorsVehicleFB : Inport  Port=7
  PantographVehicleFB : Inport  Port=8
  BrakesVehicleFB : Inport  Port=9
  DynamicsVehicleFB : Inport  Port=10
  TCMSInputAdapter : BEML_EMU_TCMSInput_Lib/TCMSInputAdapter  SystemSampleTime=ElectricalSampleTime  Latency=0  AutoFrameSizeCalculation=off
  TCMSSystem : ModelReference  ModelNameDialog=TCMSSystem  ParameterArgumentNames=Prm_TCMSSystem  ParameterArgumentValues=PRM_SimIntegration.TCMS  UsingDefaultArgumentValue=0  SimulationMode=Normal  ModelReferenceVersion=1.2279
  TCMSVehicleOut : Outport  VectorParamsAs1DForOutWhenUnconnected=off
  wires:
  ElectricalVehicleFB/1 -> TCMSInputAdapter/7
  PantographVehicleFB/1 -> TCMSInputAdapter/11
  DoorsVehicleFB/1 -> TCMSInputAdapter/10
  In Bus Element3/1 -> TCMSInputAdapter/4
  TractionVehicleFB/1 -> TCMSInputAdapter/8
  In Bus Element1/1 -> TCMSInputAdapter/2
  In Bus Element2/1 -> TCMSInputAdapter/3
  In Bus Element4/1 -> TCMSInputAdapter/5
  TCMSInputAdapter/3 -> TCMSSystem/3
  In Bus Element/1 -> TCMSInputAdapter/1
  TCMSInputAdapter/1 -> TCMSSystem/1
  TCMSInputAdapter/5 -> TCMSSystem/5
  TCMSInputAdapter/4 -> TCMSSystem/4
  TCMSInputAdapter/2 -> TCMSSystem/2
  PneumaticsVehicleFB/1 -> TCMSInputAdapter/9
  CouplingVehicleOut/1 -> TCMSInputAdapter/6
  TCMSSystem/1 -> TCMSVehicleOut/1
  CBTCVehicleOut/1 -> TCMSInputAdapter/12
  BrakesVehicleFB/1 -> TCMSInputAdapter/13
  TCMSInputAdapter/6 -> TCMSSystem/6
  DynamicsVehicleFB/1 -> TCMSInputAdapter/14

== system BEML_EMU/BEML_EMU/TractionInterface ==
  In Bus Element : Inport  PortName=ProcessedInputs  Element=ProcessedVehicleConfig
  In Bus Element1 : Inport  PortName=ProcessedInputs  Element=ProcessedTrainInput
  In Bus Element2 : Inport  PortName=ProcessedInputs  Element=ProcessedVehicleInput
  In Bus Element4 : Inport  PortName=ProcessedInputs  Element=VehicleModelFaults
  ElectricalVehicleOut : Inport  Port=2
  TCMSVehicleOut : Inport  Port=3
  DynamicsVehicleFB : Inport  Port=4
  TractionInputAdapter : BEML_EMU_TractionInput_Lib/TractionInputAdapter  SystemSampleTime=TractionSampleTime  Latency=0  AutoFrameSizeCalculation=off
  TractionSystem : ModelReference  ModelNameDialog=TractionSystem  ParameterArgumentNames=Prm_TractionSystem  ParameterArgumentValues=PRM_SimIntegration.Traction  UsingDefaultArgumentValue=0  SimulationMode=Normal  ModelReferenceVersion=1.675
  TractionVehicleOut : Outport  VectorParamsAs1DForOutWhenUnconnected=off
  wires:
  TractionSystem/1 -> TractionVehicleOut/1
  ElectricalVehicleOut/1 -> TractionInputAdapter/5
  DynamicsVehicleFB/1 -> TractionInputAdapter/7
  TractionInputAdapter/2 -> TractionSystem/2
  TractionInputAdapter/4 -> TractionSystem/4
  TractionInputAdapter/5 -> TractionSystem/5
  TractionInputAdapter/1 -> TractionSystem/1
  In Bus Element/1 -> TractionInputAdapter/1
  TractionInputAdapter/3 -> TractionSystem/3
  In Bus Element4/1 -> TractionInputAdapter/4
  In Bus Element2/1 -> TractionInputAdapter/3
  In Bus Element1/1 -> TractionInputAdapter/2
  TCMSVehicleOut/1 -> TractionInputAdapter/6

== system BEML_EMU/InputsInterface/FaultHandler ==
  VehicleConfig : Inport
  TrainInput : Inport  Port=2
  VehicleInput : Inport  Port=3
  InputControlsStates : Inport  Port=4
  PneumaticSystemFB : Inport  Port=5
  TCMSSystemFB : Inport  Port=6
  Bus Selector2 : BusSelector  OutputSignals=Faults
  Subsystem : Subsystem
  IOControlsModelFaults : Outport  VectorParamsAs1DForOutWhenUnconnected=off
  VehicleModelFaults : Outport  Port=2  VectorParamsAs1DForOutWhenUnconnected=off
  TrainFaultStates : Outport  Port=3  VectorParamsAs1DForOutWhenUnconnected=off
  VehicleFaultStates : Outport  Port=4  VectorParamsAs1DForOutWhenUnconnected=off
  wires:
  VehicleConfig/1 -> Subsystem/1(VehicleConfig)
  TrainInput/1 -> Bus Selector2/1
  VehicleInput/1 -> Subsystem/3(VehicleInput)
  InputControlsStates/1 -> Subsystem/4(InputControlStates)
  Subsystem/1(IOControlsModelFaults) -> IOControlsModelFaults/1
  Subsystem/2(VehicleModelFaults) -> VehicleModelFaults/1
  Subsystem/3(VehicleFaultStates) -> VehicleFaultStates/1
  Bus Selector2/1 -> TrainFaultStates/1, Subsystem/2(TrainFaults)  "<Faults>"
  PneumaticSystemFB/1 -> Subsystem/5(PneumaticSystemFB)
  TCMSSystemFB/1 -> Subsystem/6(TCMSSystemFB)

== system BEML_EMU/InputsInterface/IOControlsInterface ==
  VehicleConfig : Inport
  TrainInput : Inport  Port=2
  VehicleInput : Inport  Port=3
  IOControlsInput : Inport  Port=4
  ElectricalFB : Inport  Port=5
  DoorSystemFB : Inport  Port=6
  IOControlFaults : Inport  Port=7
  For Each Subsystem : Subsystem  TreatAsAtomicUnit=on
  IOControlsModel : ModelReference  ModelNameDialog=IOControls  SimulationMode=Normal  ModelReferenceVersion=1.62
  InhibitsAndInternalRequests : Subsystem
  Terminator : Terminator
  Unit Delay : UnitDelay  SampleTime=-1  HasFrameUpgradeWarning=on
  InputControlStates : Outport  VectorParamsAs1DForOutWhenUnconnected=off
  IOControlSystemOut : Outport  Port=2  VectorParamsAs1DForOutWhenUnconnected=off
  wires:
  For Each Subsystem/1(InputControlStates) -> Unit Delay/1, InputControlStates/1
  IOControlsModel/1 -> For Each Subsystem/1(IOControlsStates), IOControlSystemOut/1
  VehicleConfig/1 -> InhibitsAndInternalRequests/1(VehicleConfig)
  TrainInput/1 -> InhibitsAndInternalRequests/2(TrainInput)
  VehicleInput/1 -> InhibitsAndInternalRequests/3(VehicleInput)
  IOControlsInput/1 -> InhibitsAndInternalRequests/4(IOControlsInput)
  IOControlFaults/1 -> InhibitsAndInternalRequests/5(IOControlFaults)
  InhibitsAndInternalRequests/1(ModelInputs) -> IOControlsModel/1
  IOControlsModel/2 -> Terminator/1
  Unit Delay/1 -> InhibitsAndInternalRequests/8(IOControlStates)
  ElectricalFB/1 -> InhibitsAndInternalRequests/6(ElectricalFB)
  DoorSystemFB/1 -> InhibitsAndInternalRequests/7(DoorSystemFB)

== system BEML_EMU/InputsInterface/TrainProcessing ==
  note: BN 11/07/22: AutoPowerOn to affect the model during initialization phase only
  TrainInputs : Inport
  ModelStatus : Inport  Port=2
  AND : Logic  AllPortsSameDT=off  OutDataTypeStr=boolean
  Bus Assignment : BusAssignment  AssignedSignals=Overrides.AutoPowerOn
  Bus Selector : BusSelector  OutputSignals=IsInitialized
  Bus Selector1 : BusSelector  OutputSignals=Overrides.AutoPowerOn
  Data Type Conversion : DataTypeConversion
  NOT : Logic  Operator=NOT  AllPortsSameDT=off  OutDataTypeStr=boolean
  ProcessedTrainInputs : Outport
  wires:
  Bus Assignment/1 -> ProcessedTrainInputs/1
  TrainInputs/1 -> Bus Selector1/1, Bus Assignment/1
  ModelStatus/1 -> Bus Selector/1
  Bus Selector/1 -> NOT/1  "<IsInitialized>"
  AND/1 -> Data Type Conversion/1
  NOT/1 -> AND/2
  Bus Selector1/1 -> AND/1  "<AutoPowerOn>"
  Data Type Conversion/1 -> Bus Assignment/2

== system BEML_EMU/InputsInterface/VehicleConfigProcessing ==
  VehicleConfig : Inport
  TrainInput : Inport  Port=2
  Step : Step  Before=1  After=0  SampleTime=ConfigSampleTime
  VehicleConfigInterface : Subsystem
  VehicleConfigProcessed : Outport  VectorParamsAs1DForOutWhenUnconnected=off
  wires:
  VehicleConfigInterface/1(VehicleConfigProcessed) -> VehicleConfigProcessed/1
  VehicleConfig/1 -> VehicleConfigInterface/1(VehicleConfig)
  TrainInput/1 -> VehicleConfigInterface/2(TrainInput)
  Step/1 -> VehicleConfigInterface/Enable

== system BEML_EMU/SimulatorSystems/AudioSystemInterface ==
  DynamicsVehicleOut1 : Inport
  TractionVehicleOut1 : Inport  Port=2
  BrakesVehicleOut1 : Inport  Port=3
  PneumaticsVehicleOut1 : Inport  Port=4
  DoorsVehicleOut1 : Inport  Port=5
  PantographVehicleOut1 : Inport  Port=6
  TCMSVehicleOut1 : Inport  Port=7
  ElectricalVehicleOut1 : Inport  Port=8
  CouplingOutput : Inport  Port=9
  Subsystem1 : Subsystem
  Terminator : Terminator
  Terminator1 : Terminator
  AudioOut : Outport
  wires:
  TractionVehicleOut1/1 -> Subsystem1/2(Traction)
  DynamicsVehicleOut1/1 -> Subsystem1/1(Dynamics)
  ElectricalVehicleOut1/1 -> Subsystem1/6(Electrical)
  PantographVehicleOut1/1 -> Subsystem1/5(Panto)
  Subsystem1/1(AudioOut) -> AudioOut/1
  BrakesVehicleOut1/1 -> Terminator/1
  DoorsVehicleOut1/1 -> Subsystem1/4(Doors)
  PneumaticsVehicleOut1/1 -> Subsystem1/3(Pneumatics)
  CouplingOutput/1 -> Subsystem1/7(CouplingOutput)
  TCMSVehicleOut1/1 -> Terminator1/1

== system BEML_EMU/SimulatorSystems/Dynamics ==
  VehicleIn : Inport  Partition=on  PartitionDimension=1  PartitionWidth=1  PartitionOffset=0
  Bus Selector : BusSelector  OutputSignals=Dynamics
  For Each : ForEach  DisableCoverage=on
  <Dynamics> : Outport  ConcatenationDimension=1
  wires:
  VehicleIn/1 -> Bus Selector/1
  Bus Selector/1 -> <Dynamics>/1  "<Dynamics>"

== system BEML_EMU/SimulatorSystems/ScoringSystemInterface ==
  DynamicsVehicleOut : Inport
  TractionVehicleOut : Inport  Port=2
  BrakesVehicleOut : Inport  Port=3
  PneumaticsVehicleOut : Inport  Port=4
  DoorsVehicleOut : Inport  Port=5
  PantographVehicleOut : Inport  Port=6
  TCMSVehicleOut : Inport  Port=7
  ElectricalVehicleOut : Inport  Port=8
  Terminator{,2,4..6} (5 alike) : Terminator
  TrainLevelScoring : Subsystem
  VehicleLevelScoring : Subsystem
  ScoringTrainOutput : Outport
  ScoringVehicleOutputs : Outport  Port=2
  wires:
  DynamicsVehicleOut/1 -> Terminator/1
  TractionVehicleOut/1 -> TrainLevelScoring/1(TractionOut)
  BrakesVehicleOut/1 -> Terminator2/1
  DoorsVehicleOut/1 -> Terminator4/1
  PantographVehicleOut/1 -> Terminator5/1
  TCMSVehicleOut/1 -> Terminator6/1
  ElectricalVehicleOut/1 -> TrainLevelScoring/2(ElectricalVehicleOut), VehicleLevelScoring/1(ElectricalOut)
  VehicleLevelScoring/1(Scoring) -> ScoringVehicleOutputs/1
  PneumaticsVehicleOut/1 -> VehicleLevelScoring/2(PneumaticsVehicleOut)
  TrainLevelScoring/1(Out1) -> ScoringTrainOutput/1

== system BEML_EMU/SimulatorSystems/Subsystem ==
  Vehicle Input : Inport
  Dynamics Input : Inport  Port=2
  DynamicsVehicleOut : Inport  Port=3
  MotionBase Inputs : Inport  Port=4
  Input Adapter : Subsystem
  MotionBaseAdaptorInterface : MotionBaseAdaptersLib/MotionBase/MotionBaseAdaptorInterface
  MotionBaseOutputs : Outport
  wires:
  MotionBaseAdaptorInterface/1 -> MotionBaseOutputs/1
  Vehicle Input/1 -> Input Adapter/1(Vehicle Input)
  Dynamics Input/1 -> Input Adapter/2(Dynamics In)
  MotionBase Inputs/1 -> Input Adapter/3(MotionBaseInputs)
  Input Adapter/1(MotionBaseInput) -> MotionBaseAdaptorInterface/1
  DynamicsVehicleOut/1 -> Input Adapter/4(DynamicsOut)

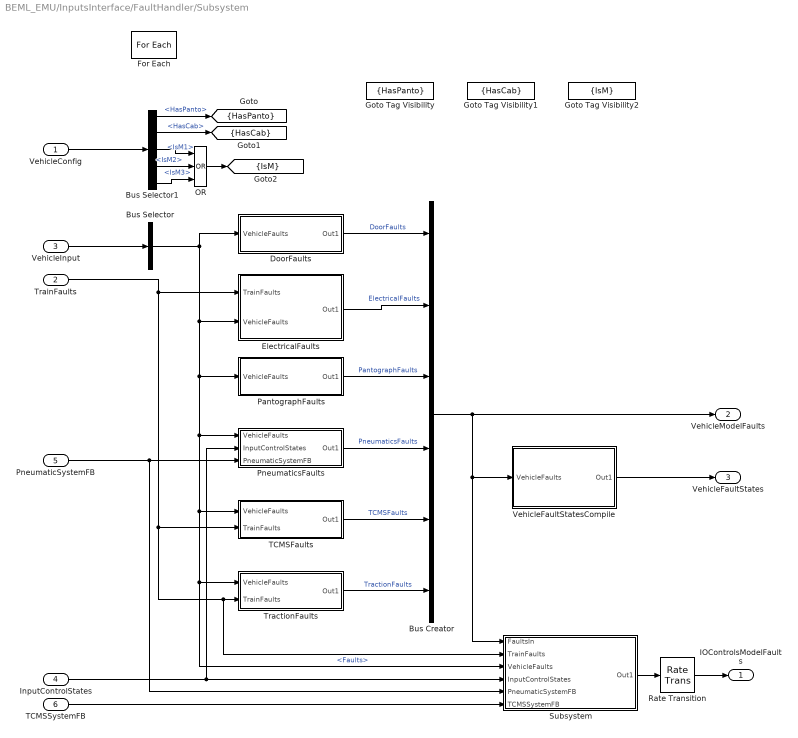
== system BEML_EMU/InputsInterface/FaultHandler/Subsystem ==
  VehicleConfig : Inport  Partition=on  PartitionDimension=1  PartitionWidth=1  PartitionOffset=0
  TrainFaults : Inport  Port=2
  VehicleInput : Inport  Port=3  Partition=on  PartitionDimension=1  PartitionWidth=1  PartitionOffset=0
  InputControlStates : Inport  Port=4  Partition=on  PartitionDimension=1  PartitionWidth=1  PartitionOffset=0
  PneumaticSystemFB : Inport  Port=5  Partition=on  PartitionDimension=1  PartitionWidth=1  PartitionOffset=0
  TCMSSystemFB : Inport  Port=6  Partition=on  PartitionDimension=1  PartitionWidth=1  PartitionOffset=0
  Bus Creator : BusCreator  Inputs=6  OutDataTypeStr=Bus: BD_SimIntegration_Faults_Vehicle_Processed  NonVirtualBus=on
  Bus Selector : BusSelector  OutputSignals=Faults
  Bus Selector1 : BusSelector  OutputSignals=Electrical.HasPanto,Electrical.HasCab,Electrical.IsM1,Electrical.IsM2,Electrical.IsM3
  DoorFaults : Subsystem
  ElectricalFaults : Subsystem
  For Each : ForEach  DisableCoverage=on
  Goto Tag Visibility : GotoTagVisibility  GotoTag=HasPanto
  Goto Tag Visibility1 : GotoTagVisibility  GotoTag=HasCab
  Goto Tag Visibility2 : GotoTagVisibility  GotoTag=IsM
  OR : Logic  Operator=OR  Inputs=3  AllPortsSameDT=off  OutDataTypeStr=boolean
  PantographFaults : Subsystem
  PneumaticsFaults : Subsystem
  Rate Transition : RateTransition
  Subsystem : Subsystem
  TCMSFaults : Subsystem
  TractionFaults : Subsystem
  VehicleFaultStatesCompile : Subsystem
  IOControlsModelFaults : Outport  ConcatenationDimension=1
  VehicleModelFaults : Outport  Port=2  ConcatenationDimension=1
  VehicleFaultStates : Outport  Port=3  ConcatenationDimension=1
  tag scope: HasCab=scoped, HasPanto=scoped, IsM=scoped
  wires:
  VehicleConfig/1 -> Bus Selector1/1
  Bus Selector/1 -> DoorFaults/1(VehicleFaults), PantographFaults/1(VehicleFaults), Subsystem/3(VehicleFaults), TractionFaults/1(VehicleFaults), TCMSFaults/1(VehicleFaults), PneumaticsFaults/1(VehicleFaults), ElectricalFaults/2(VehicleFaults)  "<Faults>"
  TractionFaults/1(Out1) -> Bus Creator/6  "TractionFaults"
  PantographFaults/1(Out1) -> Bus Creator/3  "PantographFaults"
  PneumaticsFaults/1(Out1) -> Bus Creator/4  "PneumaticsFaults"
  ElectricalFaults/1(Out1) -> Bus Creator/2  "ElectricalFaults"
  TCMSFaults/1(Out1) -> Bus Creator/5  "TCMSFaults"
  DoorFaults/1(Out1) -> Bus Creator/1  "DoorFaults"
  VehicleFaultStatesCompile/1(Out1) -> VehicleFaultStates/1
  VehicleInput/1 -> Bus Selector/1
  Bus Selector1/1 -> [HasPanto]  "<HasPanto>"
  TrainFaults/1 -> TCMSFaults/2(TrainFaults), Subsystem/2(TrainFaults), TractionFaults/2(TrainFaults), ElectricalFaults/1(TrainFaults)
  Rate Transition/1 -> IOControlsModelFaults/1
  Bus Selector1/2 -> [HasCab]  "<HasCab>"
  Subsystem/1(Out1) -> Rate Transition/1
  Bus Selector1/4 -> OR/2  "<IsM2>"
  Bus Selector1/3 -> OR/1  "<IsM1>"
  Bus Selector1/5 -> OR/3  "<IsM3>"
  OR/1 -> [IsM]
  Bus Creator/1 -> VehicleModelFaults/1, Subsystem/1(FaultsIn), VehicleFaultStatesCompile/1(VehicleFaults)
  PneumaticSystemFB/1 -> Subsystem/5(PneumaticSystemFB), PneumaticsFaults/3(PneumaticSystemFB)
  TCMSSystemFB/1 -> Subsystem/6(TCMSSystemFB)
  InputControlStates/1 -> PneumaticsFaults/2(InputControlStates), Subsystem/4(InputControlStates)

== system BEML_EMU/InputsInterface/IOControlsInterface/For Each Subsystem ==
  IOControlsStates : Inport  Partition=on  PartitionDimension=1  PartitionWidth=1  PartitionOffset=0
  Bus Selector : BusSelector  OutputSignals=InputStates
  For Each : ForEach  DisableCoverage=on
  InputControlStates : Outport  ConcatenationDimension=1
  wires:
  IOControlsStates/1 -> Bus Selector/1
  Bus Selector/1 -> InputControlStates/1  "<InputStates>"
